simulink model "vehicle_motion_model_final_temp"  (R2021b)
settings: Solver=ode5  StartTime=0.0  StopTime=600  FixedStep=0.001  RelTol=1e-3
StopFcn:
  | % stop simulation callback function
  | figure(1);
  | out.x_gt.data = permute(out.x_gt.data,[3, 1, 2]);
  | plot3(out.x_gt.data(:, 1), out.x_gt.data(:, 2), -out.x_gt.data(:, 3), 'Color', 'r', 'LineWidth', 1.5);
  | legend('Истинная траектория')
  | xlabel('X, \itм');
  | ylabel('Y, \itм');
  | zlabel('Z, \itм');
  | figure(2);
  | plot3(out.x.data(:, 1), out.x.data(:, 2), -out.x.data(:, 3), 'Color', 'b', 'LineWidth', 1.5);
  | hold on;
  | xlabel('X, \itм');
  | ylabel('Y, \itм');
  | zlabel('Z, \itм');
  | % legend('pos')
  | hold on;
  | plot3(out.x_gt.data(:, 1), out.x_gt.data(:, 2), -out.x_gt.data(:, 3), 'Color', 'r', 'LineWidth', 1.5);
  | hold on;
  | legend('Рассчитанная траектория', 'Истинная траектория')
  | % errors
  | figure(3);
  | yyaxis left;
  | plot(out.hor_err_fus.time, out.hor_err_fus.data, 'Color', 'b', 'LineWidth', 1.5);
  | xlabel('время, \itс');
  | ylabel('Горизонтальная ошибка, \itм');
  | hold on;
  | yyaxis right;
  | plot(out.ver_err_fus.time, out.ver_err_fus.data, 'Color', 'r', 'LineWidth', 1.5);
  | ylabel('Вертикальная ошибка, \itм');
  | legend('Горизонтальная позиционная ошибка', 'Вертикальная позиционная ошибка');
  | grid on;
  | figure(4);
  | yyaxis left;
  | plot(out.hor_err_ins.time, out.hor_err_ins.data, '-', 'Color', 'b', 'LineWidth', 1.5);
  | xlabel('время, \itс');
  | ylabel('Горизонтальная ошибка, \itм');
  | hold on;
  | yyaxis right;
  | plot(out.ver_err_ins.time, out.ver_err_ins.data, '-', 'Color', 'r', 'LineWidth', 1.5);
  | ylabel('Вертикальная ошибка, \itм');
  | legend('Горизонтальная позиционная ошибка', 'Вертикальная позиционная ошибка');
  | grid on;
model workspace (MAT data in the model file):
  AxlIxx = 62.3745166667
  AxlM = 160
  Cps = 2
  CzWhlAxl = 557955.087061
  DCT_Param : object (value not decoded)
  Downshift_Speeds = [9.5625 12.9375 16.3125 19.6875 23.0625 26.4375 29.8125 33.1875 36.5625 39.9375 43.3125 46.6875 ... (28 elements, 4x7)]
  F0zWhlAxl = 16132.2380068
  HTCH : object (value not decoded)
  Hmax = 0.25
  KzWhlAxl = 58428920.0848
  NCyl = 6
  Pedal_Positions = [0.1 0.4 0.5 0.9]
  Pstd = 101325
  Q = [1  0  0; 0  1  0; 0  0  1]
  Rair = 287
  SUS : object (value not decoded)
  TRA : object (value not decoded)
  Trans : object (value not decoded)
  Tstd = 293.15
  Upshift_Speeds = [12.9375 16.3125 19.6875 33 26.4375 29.8125 33.1875 52.5 39.9375 43.3125 46.6875 77.25 ... (28 elements, 4x7)]
  VEH : object (value not decoded)
  Vd = 0.00346
  WH : Mass (value not decoded)
  dt3D = 0.05
  f_air = [0 0 0 0 0 0 0 0 0 0 0 0 ... (256 elements, 16x16)]
  f_co = [0 0 0 0 0 0 0 0 0 0 0 0 ... (256 elements, 16x16)]
  f_co2 = [0 0 0 0 0 0 0 0 0 0 0 0 ... (256 elements, 16x16)]
  f_eff = [352.135682859 352.135682859 320.724378192 303.655312657 295.930136708 291.240087194 291.240271258 291.240312459 291.240275452 291.240198499 291.240100781 291.240018769 ... (256 elements, 16x16)]
  f_fuel = [0 0 0 0 0 0 0 0 0 0 0 0 ... (256 elements, 16x16)]
  f_hc = [0 0 0 0 0 0 0 0 0 0 0 0 ... (256 elements, 16x16)]
  f_nox = [0 0 0 0 0 0 0 0 0 0 0 0 ... (256 elements, 16x16)]
  f_pm = [0 0 0 0 0 0 0 0 0 0 0 0 ... (256 elements, 16x16)]
  f_susp_axl_bp = [1 2]
  f_susp_dz_bp = [-0.325022776267 -0.315022776267 -0.305022776267 -0.205022776267 -0.105022776267 -0.00502277626717 0.0949772237328 0.194977223733 0.204977223733 0.214977223733]
  f_susp_dzdot_bp = [-3 -0.3 -0.2 -0.1 0 0.1 0.2 0.3 3]
  f_susp_fmz = [-144070.391448 -93629.24037 -75929.1118915 -20630.5828179 -15385.48216 -10140.3815021 -4895.28084414 349.819813785 -31916.3973792 18437.6709544 -83996.1993354 -33555.0482577 ... (43920 elements, 10x9x61x2x4)]
  f_susp_geom = [0 0 0 0 0 0 0 0 0 0 0 0 ... (3660 elements, 10x61x2x3)]
  f_susp_strgdelta_bp = [-0.523598775598 -0.506145483078 -0.488692190558 -0.471238898038 -0.453785605519 -0.436332312999 -0.418879020479 -0.401425727959 -0.383972435439 -0.366519142919 -0.349065850399 -0.331612557879 ... (61 elements, 1x61)]
  f_tbrake = [0 76.8593923996 105.140482948 131.533638111 157.926793274 176.658631717 176.65727296 176.656856686 176.656879077 176.657093756 176.657404516 176.65772406 ... (256 elements, 16x16)]
  f_tbrake_n_bpt = [0 649.519052838 912.419621844 1175.32019085 1438.22075986 1701.12132886 1964.02189787 2226.92246687 2489.82303588 2752.72360489 3015.62417389 3278.5247429 ... (16 elements, 1x16)]
  f_tbrake_t_bpt = [0 34.6410161514 61.0341713143 87.4273264773 113.82048164 140.213636803 166.606791966 192.999947129 219.393102292 245.786257455 272.179412618 298.572567781 ... (16 elements, 1x16)]
  f_texh = [766.752464599 766.752464599 786.17542386 801.679939032 884.591982581 910.574397722 910.571871054 910.570774534 910.570601632 910.570821151 910.571247242 910.571639815 ... (256 elements, 16x16)]
  f_twc_eff_co = [0.17 0.25 0.45 0.99 0.99 0.99 0.99]
  f_twc_eff_hc = [0.21 0.375 0.75 0.98 0.98 0.98 0.98]
  f_twc_eff_lam = [0.909090909 0.944055944 0.979020979 1 1.013986014 1.048951049 1.083916084]
  f_twc_eff_nox = [0.98 0.98 0.98 0.97 0.05 0.02 0]
  h = 0.134
symbols that are objects in the model workspace (value not decoded): VEH
libraries: aerolibcommonsys x8, sharedtransform x8, sharedutil x7, autolibsharedcommon x7, autolibutils x4, vehdynlibtirecommon x3, dspstat3 x2, mspsensorlib x1, aerolibnav x1, shared6dof x1, autolibshared x1, vehdynlibsuspension x1
(part 5 of 9)

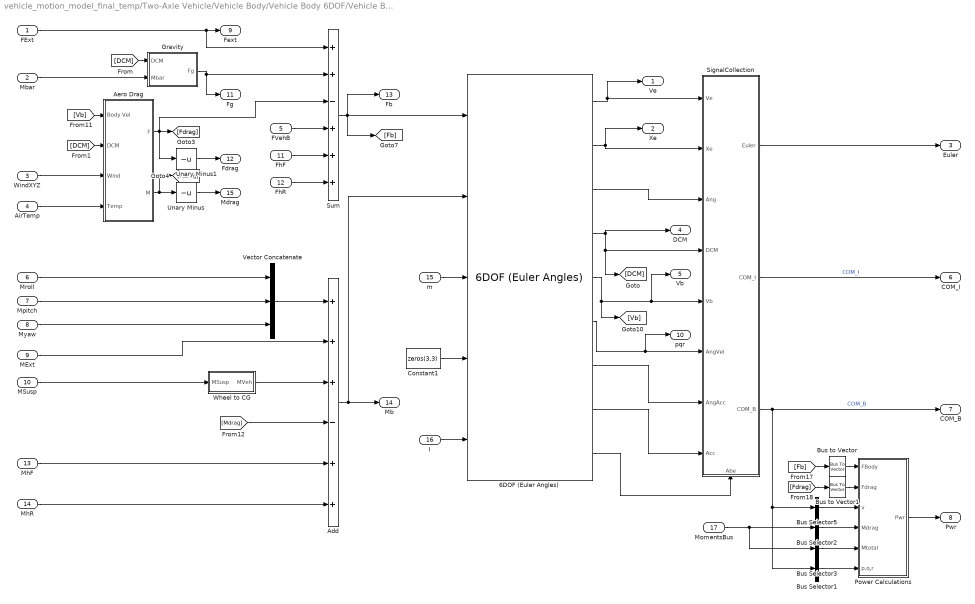
== system vehicle_motion_model_final_temp/Two-Axle Vehicle/Vehicle Body/Vehicle Body 6DOF/Vehicle Body 6DOF/6 DOF Generic Vehicle Body ==
  FExt : Inport  Unit=N
  Mbar : Inport  Port=2
  WindXYZ : Inport  Port=3  Unit=m/s
  AirTemp : Inport  Port=4  Unit=K
  FVehB : Inport  Port=5
  Mroll : Inport  Port=6
  Mpitch : Inport  Port=7
  Myaw : Inport  Port=8
  MExt : Inport  Port=9  Unit=N*m
  MSusp : Inport  Port=10  Unit=N*m
  FhF : Inport  Port=11  Unit=N
  FhR : Inport  Port=12  Unit=N
  MhF : Inport  Port=13  Unit=N*m
  MhR : Inport  Port=14  Unit=N*m
  m : Inport  Port=15
  I : Inport  Port=16
  MomentsBus : Inport  Port=17  Unit=N*m
  6DOF (Euler Angles) : shared6dof/6DOF (Euler Angles)  units=Metric (MKS)  mtype=Custom Variable  rep=Euler Angles  xme_0=Xe_o  Vm_0=xbdot_o  eul_0=eul_o  pm_0=p_o  mass_0=m  mass_e=[0 0 0]  mass_f=[0 0 0]  inertia=Iveh  inertia_e=[0 0 0]  inertia_f=[0 0 0]  k_quat=[0 0 0]  vre_flag=off  abi_flag=on  aMode=2  xme_statename=''  Vm_statename=''  eul_statename=''  quat_statename=''  pm_statename=''  mass_statename=''
      settings: SourceProductBaseCode=AE,PW,DR,MT,UV,VE
  Add : Sum  Inputs=+++-++
  Aero Drag : Subsystem
  Bus Selector1 : BusSelector  OutputSignals=AngVel.p,AngVel.q,AngVel.r  OutputAsBus=on
  Bus Selector2 : BusSelector  OutputSignals=Drag.Mx,Drag.My,Drag.Mz  OutputAsBus=on
  Bus Selector3 : BusSelector  OutputSignals=Body.Mx,Body.My,Body.Mz  OutputAsBus=on
  Bus Selector5 : BusSelector  OutputSignals=Vel.xdot,Vel.ydot,Vel.zdot  OutputAsBus=on
  Bus to Vector : BusToVector
  Bus to Vector1 : BusToVector
  Constant1 : Constant  Value=zeros(3,3)
  Gravity : Subsystem
  Power Calculations : Subsystem  VariantControl=2
  SignalCollection : Subsystem
      settings: PortSchema="{\"entries\":[{\"content\":{\"sides\":[{\"content\":{\"connectorIds\":[\"In1\",\"In2\",\"In3\",\"In4\",\"In5\",\"In6\",\"In7\",\"In8\"]},\"type\":\"ConnectorPlacement.EquallySpacedRectSide\",\"uuid\":\"876487b8-56e9-4112-b104-05c1a2771af8\"},{\"content\":{\"connectorIds\":[\"Out1\",\"Out2\",\"Out3\"],\"side\":\"RIGHT\"},\"type\":\"ConnectorPlacement.EquallySpacedRectSide\",\"uuid\":\"0e979842-5463-4993-8b9a-4ed5d1e46013\"},{\"content\":{\"connectorIds\":[],\"side\":\"TOP\"},\"type\":\"ConnectorPlacement.EquallySpacedRectSide\",\"uuid\":\"9909ba18-debd-4c28-8048-279359011dab\"},{\"content\":{\"connectorIds\":[\"In9\"],\"side\":\"BOTTOM\"},\"type\":\"ConnectorPlacement.EquallySpacedRectSide\",\"uuid\":\"e172f998-bdb6-4b24-8333-70df8a68a329\"}]},\"type\":\"ConnectorPlacement.EquallySpacedConnector\",\"uuid\":\"1f4bc3e0-d188-4108-8b40-be3dce1f4c41\"}],\"packageUris\":[\"http://schema.mathworks.com/mf0/Connector/R2020b\"],\"version\":\"1.0\"}"
  Sum : Sum  Inputs=++-+++  InputSameDT=on  SaturateOnIntegerOverflow=on  OutDataTypeStr=Inherit: Same as first input
  Unary Minus : UnaryMinus
  Unary Minus1 : UnaryMinus
  Vector Concatenate : Concatenate  NumInputs=3
  Wheel to CG : Subsystem
  Ve : Outport  Unit=m/s  VectorParamsAs1DForOutWhenUnconnected=off
  Xe : Outport  Port=2  Unit=m  VectorParamsAs1DForOutWhenUnconnected=off
  Euler : Outport  Port=3  Unit=rad  VectorParamsAs1DForOutWhenUnconnected=off
  DCM : Outport  Port=4  VectorParamsAs1DForOutWhenUnconnected=off
  Vb : Outport  Port=5  Unit=m/s  VectorParamsAs1DForOutWhenUnconnected=off
  COM_I : Outport  Port=6  VectorParamsAs1DForOutWhenUnconnected=off
  COM_B : Outport  Port=7  VectorParamsAs1DForOutWhenUnconnected=off
  Pwr : Outport  Port=8  VectorParamsAs1DForOutWhenUnconnected=off
  Fext : Outport  Port=9  VectorParamsAs1DForOutWhenUnconnected=off
  pqr : Outport  Port=10  Unit=rad/s  VectorParamsAs1DForOutWhenUnconnected=off
  Fg : Outport  Port=11  VectorParamsAs1DForOutWhenUnconnected=off
  Fdrag : Outport  Port=12  VectorParamsAs1DForOutWhenUnconnected=off
  Fb : Outport  Port=13  VectorParamsAs1DForOutWhenUnconnected=off
  Mb : Outport  Port=14  VectorParamsAs1DForOutWhenUnconnected=off
  Mdrag : Outport  Port=15  VectorParamsAs1DForOutWhenUnconnected=off
  wires:
  6DOF (Euler Angles)/9 -> SignalCollection/9(Abe)
  Unary Minus1/1 -> Fdrag/1
  Unary Minus/1 -> Mdrag/1
  MomentsBus/1 -> Bus Selector2/1, Bus Selector3/1
  MhR/1 -> Add/6
  FhR/1 -> Sum/6
  FhF/1 -> Sum/5
  MhF/1 -> Add/5
  Mbar/1 -> Gravity/2(Mbar)
  I/1 -> 6DOF (Euler Angles)/5
  Mpitch/1 -> Vector Concatenate/2
  Myaw/1 -> Vector Concatenate/3
  Bus Selector3/1 -> Power Calculations/5(Mtotal)
  SignalCollection/1(Euler) -> Euler/1
  [Mdrag] -> Add/4
  Bus to Vector/1 -> Power Calculations/1(FBody)
  Power Calculations/1(Pwr) -> Pwr/1
  6DOF (Euler Angles)/2 -> Xe/1, SignalCollection/2(Xe)
  AirTemp/1 -> Aero Drag/4(Temp)
  [Fdrag] -> Bus to Vector1/1
  Vector Concatenate/1 -> Add/1
  MExt/1 -> Add/2
  6DOF (Euler Angles)/6 -> SignalCollection/6(AngVel), pqr/1
  6DOF (Euler Angles)/5 -> SignalCollection/5(Vb), Vb/1, [Vb]
  FExt/1 -> Fext/1, Sum/1
  6DOF (Euler Angles)/4 -> DCM/1, SignalCollection/4(DCM), [DCM]
  MSusp/1 -> Wheel to CG/1(MSusp)
  FVehB/1 -> Sum/4
  [DCM] -> Aero Drag/2(DCM)
  SignalCollection/2(COM_I) -> COM_I/1  "COM_I"
  WindXYZ/1 -> Aero Drag/3(Wind)
  [Vb] -> Aero Drag/1(Body Vel)
  Gravity/1(Fg) -> Sum/2, Fg/1
  [DCM] -> Gravity/1(DCM)
  Aero Drag/2(M) -> [Mdrag], Unary Minus/1
  6DOF (Euler Angles)/3 -> SignalCollection/3(Ang)
  Bus Selector5/1 -> Power Calculations/3(v)
  Sum/1 -> 6DOF (Euler Angles)/1, [Fb], Fb/1
  Mroll/1 -> Vector Concatenate/1
  6DOF (Euler Angles)/8 -> SignalCollection/8(Acc)
  Wheel to CG/1(MVeh) -> Add/3
  6DOF (Euler Angles)/7 -> SignalCollection/7(AngAcc)
  Bus to Vector1/1 -> Power Calculations/2(Fdrag)
  m/1 -> 6DOF (Euler Angles)/3
  [Fb] -> Bus to Vector/1
  SignalCollection/3(COM_B) -> Bus Selector5/1, Bus Selector1/1, COM_B/1  "COM_B"
  Add/1 -> Mb/1, 6DOF (Euler Angles)/2
  6DOF (Euler Angles)/1 -> Ve/1, SignalCollection/1(Ve)
  Constant1/1 -> 6DOF (Euler Angles)/4
  Bus Selector2/1 -> Power Calculations/4(Mdrag)
  Bus Selector1/1 -> Power Calculations/6(p,q,r)
  Aero Drag/1(F) -> Sum/3, [Fdrag], Unary Minus1/1

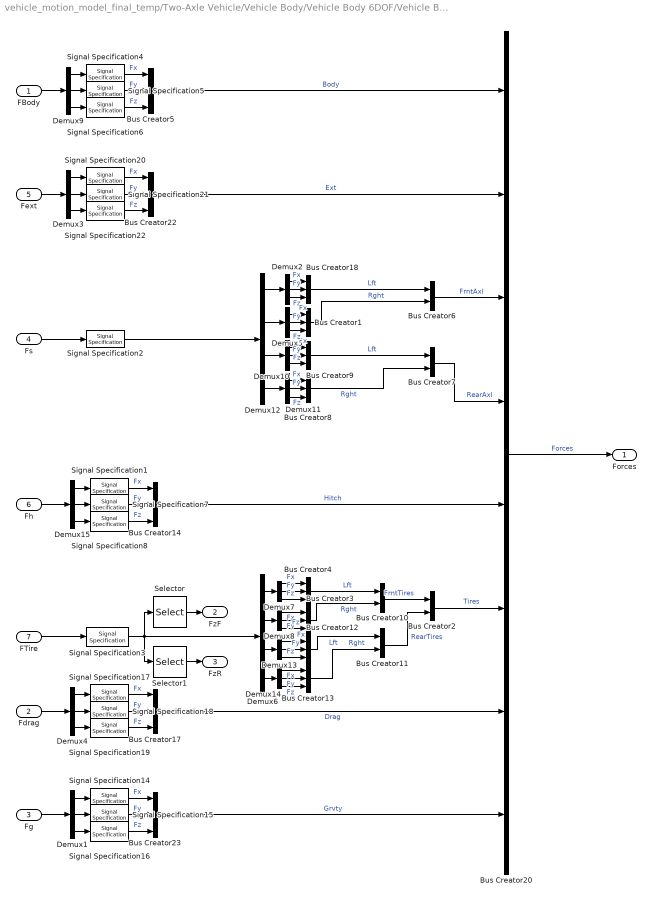
== system vehicle_motion_model_final_temp/Two-Axle Vehicle/Vehicle Body/Vehicle Body 6DOF/Vehicle Body 6DOF/Forces ==
  FBody : Inport
  Fdrag : Inport  Port=2
  Fg : Inport  Port=3
  Fs : Inport  Port=4  Unit=N
  Fext : Inport  Port=5
  Fh : Inport  Port=6
  FTire : Inport  Port=7
  Bus Creator{1,3..5,8..9,12..14,17..18,22..23} (13 alike) : BusCreator  Inputs=3
  Bus Creator{2,6..7,10..11} (5 alike) : BusCreator  Inputs=2
  Bus Creator20 : BusCreator  Inputs=8
  Demux{1..5,7..11,13..15} (13 alike) : Demux  Outputs=3
  Demux12 : Demux  Outputs=[3,3,3,3]
  Demux6 : Demux  Outputs=[3,3,3,3]
  Selector : Selector  InputPortWidth=12  IndexOptions=Index vector (dialog)  Indices=[3,6]  OutputSizes=1
  Selector1 : Selector  InputPortWidth=12  IndexOptions=Index vector (dialog)  Indices=[9,12]  OutputSizes=1
  Signal Specification{1..8,14..22} (17 alike) : SignalSpecification  Unit=N
  Forces : Outport  VectorParamsAs1DForOutWhenUnconnected=off
  FzF : Outport  Port=2  VectorParamsAs1DForOutWhenUnconnected=off
  FzR : Outport  Port=3  VectorParamsAs1DForOutWhenUnconnected=off
  wires:
  Bus Creator14/1 -> Bus Creator20/5  "Hitch"
  Fh/1 -> Demux15/1
  Demux15/3 -> Signal Specification8/1
  Demux15/2 -> Signal Specification7/1
  Demux15/1 -> Signal Specification1/1
  Signal Specification7/1 -> Bus Creator14/2  "Fy"
  Signal Specification1/1 -> Bus Creator14/1  "Fx"
  Signal Specification8/1 -> Bus Creator14/3  "Fz"
  Selector1/1 -> FzR/1
  Selector/1 -> FzF/1
  Demux13/3 -> Bus Creator12/3  "Fz"
  Bus Creator13/1 -> Bus Creator11/2  "Rght"
  Demux14/1 -> Bus Creator13/1  "Fx"
  Demux14/2 -> Bus Creator13/2  "Fy"
  Demux14/3 -> Bus Creator13/3  "Fz"
  Demux6/4 -> Demux14/1
  Demux6/3 -> Demux13/1
  Demux13/2 -> Bus Creator12/2  "Fy"
  Demux13/1 -> Bus Creator12/1  "Fx"
  Signal Specification2/1 -> Demux12/1
  Bus Creator12/1 -> Bus Creator11/1  "Lft"
  Bus Creator3/1 -> Bus Creator10/2  "Rght"
  Bus Creator4/1 -> Bus Creator10/1  "Lft"
  Demux12/3 -> Demux10/1
  Demux12/4 -> Demux11/1
  Demux11/1 -> Bus Creator8/1  "Fx"
  Demux11/2 -> Bus Creator8/2  "Fy"
  Demux11/3 -> Bus Creator8/3  "Fz"
  Demux10/3 -> Bus Creator9/3  "Fz"
  Demux10/2 -> Bus Creator9/2  "Fy"
  Demux10/1 -> Bus Creator9/1  "Fx"
  Bus Creator9/1 -> Bus Creator7/1  "Lft"
  Bus Creator8/1 -> Bus Creator7/2  "Rght"
  Bus Creator1/1 -> Bus Creator6/2  "Rght"
  Bus Creator18/1 -> Bus Creator6/1  "Lft"
  Demux1/1 -> Signal Specification14/1
  Fg/1 -> Demux1/1
  Demux1/3 -> Signal Specification16/1
  Demux1/2 -> Signal Specification15/1
  Bus Creator23/1 -> Bus Creator20/8  "Grvty"
  Bus Creator20/1 -> Forces/1  "Forces"
  Signal Specification16/1 -> Bus Creator23/3  "Fz"
  Signal Specification19/1 -> Bus Creator17/3  "Fz"
  Signal Specification14/1 -> Bus Creator23/1  "Fx"
  Signal Specification17/1 -> Bus Creator17/1  "Fx"
  Signal Specification18/1 -> Bus Creator17/2  "Fy"
  Signal Specification21/1 -> Bus Creator22/2  "Fy"
  Signal Specification15/1 -> Bus Creator23/2  "Fy"
  Signal Specification20/1 -> Bus Creator22/1  "Fx"
  Signal Specification22/1 -> Bus Creator22/3  "Fz"
  Bus Creator22/1 -> Bus Creator20/2  "Ext"
  Fext/1 -> Demux3/1
  Demux3/1 -> Signal Specification20/1
  Demux3/2 -> Signal Specification21/1
  Demux3/3 -> Signal Specification22/1
  Demux4/1 -> Signal Specification17/1
  Demux4/2 -> Signal Specification18/1
  Demux4/3 -> Signal Specification19/1
  Fdrag/1 -> Demux4/1
  Bus Creator6/1 -> Bus Creator20/3  "FrntAxl"
  Bus Creator7/1 -> Bus Creator20/4  "RearAxl"
  Demux2/1 -> Bus Creator18/1  "Fx"
  Demux2/2 -> Bus Creator18/2  "Fy"
  Demux2/3 -> Bus Creator18/3  "Fz"
  Demux5/3 -> Bus Creator1/3  "Fz"
  Demux5/2 -> Bus Creator1/2  "Fy"
  Demux8/1 -> Bus Creator3/1  "Fx"
  Demux8/2 -> Bus Creator3/2  "Fy"
  Demux8/3 -> Bus Creator3/3  "Fz"
  Demux7/3 -> Bus Creator4/3  "Fz"
  Demux7/2 -> Bus Creator4/2  "Fy"
  Demux7/1 -> Bus Creator4/1  "Fx"
  Bus Creator11/1 -> Bus Creator2/2  "RearTires"
  Bus Creator10/1 -> Bus Creator2/1  "FrntTires"
  Demux5/1 -> Bus Creator1/1  "Fx"
  Fs/1 -> Signal Specification2/1
  Demux12/2 -> Demux5/1
  Demux12/1 -> Demux2/1
  FTire/1 -> Signal Specification3/1
  Signal Specification3/1 -> Demux6/1, Selector/1, Selector1/1
  Demux6/1 -> Demux7/1
  Demux6/2 -> Demux8/1
  Bus Creator2/1 -> Bus Creator20/6  "Tires"
  Bus Creator17/1 -> Bus Creator20/7  "Drag"
  Bus Creator5/1 -> Bus Creator20/1  "Body"
  Demux9/3 -> Signal Specification6/1
  Demux9/2 -> Signal Specification5/1
  Demux9/1 -> Signal Specification4/1
  FBody/1 -> Demux9/1
  Signal Specification6/1 -> Bus Creator5/3  "Fz"
  Signal Specification4/1 -> Bus Creator5/1  "Fx"
  Signal Specification5/1 -> Bus Creator5/2  "Fy"

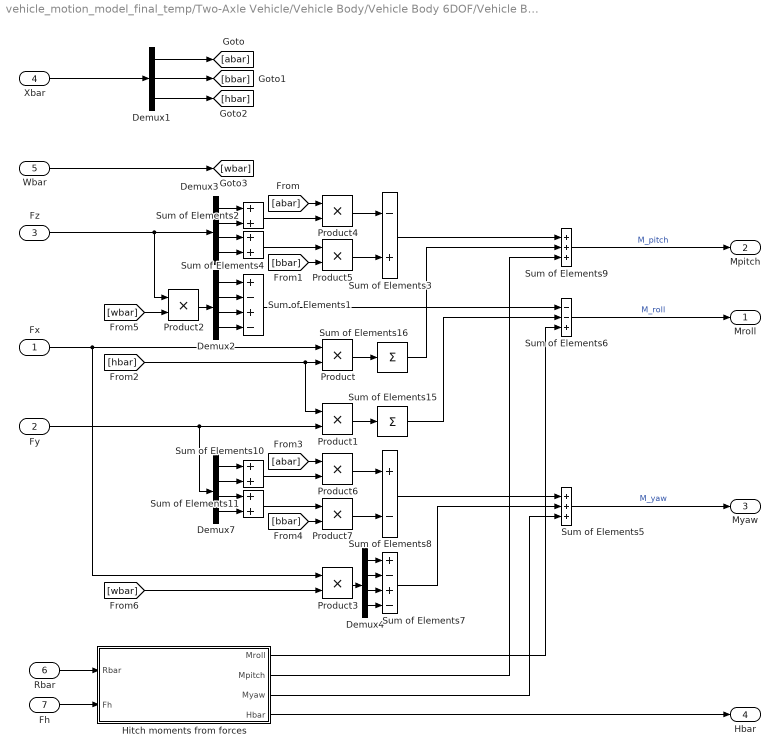
== system vehicle_motion_model_final_temp/Two-Axle Vehicle/Vehicle Body/Vehicle Body 6DOF/Vehicle Body 6DOF/Moment Calc ==
  Fx : Inport
  Fy : Inport  Port=2
  Fz : Inport  Port=3
  Xbar : Inport  Port=4
  Wbar : Inport  Port=5
  Rbar : Inport  Port=6
  Fh : Inport  Port=7
  Demux1 : Demux  Outputs=3
  Demux{2..4,7} (4 alike) : Demux
  Hitch moments from forces : Subsystem
  Product{,1..7} (8 alike) : Product
  Sum of Elements1 : Sum  Inputs=+-+-
  Sum of Elements{2,4,10..11} (4 alike) : Sum
  Sum of Elements15 : Sum  Inputs=+
  Sum of Elements16 : Sum  Inputs=+
  Sum of Elements3 : Sum  Inputs=-+
  Sum of Elements5 : Sum  Inputs=+++
  Sum of Elements6 : Sum  Inputs=--+
  Sum of Elements7 : Sum  Inputs=+-+-
  Sum of Elements8 : Sum  Inputs=+-
  Sum of Elements9 : Sum  Inputs=+++
  Mroll : Outport  VectorParamsAs1DForOutWhenUnconnected=off
  Mpitch : Outport  Port=2  VectorParamsAs1DForOutWhenUnconnected=off
  Myaw : Outport  Port=3  VectorParamsAs1DForOutWhenUnconnected=off
  Hbar : Outport  Port=4  VectorParamsAs1DForOutWhenUnconnected=off
  wires:
  Hitch moments from forces/4(Hbar) -> Hbar/1
  Fh/1 -> Hitch moments from forces/2(Fh)
  Hitch moments from forces/3(Myaw) -> Sum of Elements5/3
  Hitch moments from forces/2(Mpitch) -> Sum of Elements9/3
  Hitch moments from forces/1(Mroll) -> Sum of Elements6/3
  Rbar/1 -> Hitch moments from forces/1(Rbar)
  Wbar/1 -> [wbar]
  Demux1/1 -> [abar]
  Demux1/2 -> [bbar]
  [wbar] -> Product2/2
  Xbar/1 -> Demux1/1
  Demux1/3 -> [hbar]
  Demux7/2 -> Sum of Elements10/2
  Demux7/1 -> Sum of Elements10/1
  Demux7/4 -> Sum of Elements11/2
  Demux7/3 -> Sum of Elements11/1
  Product6/1 -> Sum of Elements8/1
  Product7/1 -> Sum of Elements8/2
  Sum of Elements11/1 -> Product7/1
  Sum of Elements10/1 -> Product6/2
  [abar] -> Product6/1
  [bbar] -> Product7/2
  [bbar] -> Product5/2
  [abar] -> Product4/1
  [wbar] -> Product3/2
  Product3/1 -> Demux4/1
  Demux4/3 -> Sum of Elements7/3
  Demux4/2 -> Sum of Elements7/2
  Product2/1 -> Demux2/1
  Demux2/3 -> Sum of Elements1/3
  Demux2/2 -> Sum of Elements1/2
  Fy/1 -> Product1/2, Demux7/1
  Demux4/1 -> Sum of Elements7/1
  Demux4/4 -> Sum of Elements7/4
  Demux2/4 -> Sum of Elements1/4
  Fx/1 -> Product/1, Product3/1
  Fz/1 -> Demux3/1, Product2/1
  Sum of Elements1/1 -> Sum of Elements6/1
  Sum of Elements2/1 -> Product4/2
  Sum of Elements4/1 -> Product5/1
  Demux3/3 -> Sum of Elements4/1
  Sum of Elements3/1 -> Sum of Elements9/1
  [hbar] -> Product/2, Product1/1
  Demux3/4 -> Sum of Elements4/2
  Demux3/1 -> Sum of Elements2/1
  Demux3/2 -> Sum of Elements2/2
  Sum of Elements15/1 -> Sum of Elements6/2
  Sum of Elements8/1 -> Sum of Elements5/1
  Sum of Elements5/1 -> Myaw/1  "M_yaw"
  Sum of Elements16/1 -> Sum of Elements9/2
  Product5/1 -> Sum of Elements3/2
  Sum of Elements7/1 -> Sum of Elements5/2
  Demux2/1 -> Sum of Elements1/1
  Product4/1 -> Sum of Elements3/1
  Sum of Elements9/1 -> Mpitch/1  "M_pitch"
  Sum of Elements6/1 -> Mroll/1  "M_roll"
  Product/1 -> Sum of Elements16/1
  Product1/1 -> Sum of Elements15/1

== system vehicle_motion_model_final_temp/Two-Axle Vehicle/Vehicle Body/Vehicle Body 6DOF/Vehicle Body 6DOF/Moments ==
  MBody : Inport
  Mdrag : Inport  Port=2
  MExt : Inport  Port=3
  Mh : Inport  Port=4
  Bus Creator{1..3,24} (4 alike) : BusCreator  Inputs=3
  Bus Creator7 : BusCreator  Inputs=4
  Demux{,1..3} (4 alike) : Demux  Outputs=3
  Signal Specification{1..11,23} (12 alike) : SignalSpecification  Unit=N*m
  Moments : Outport  VectorParamsAs1DForOutWhenUnconnected=off
  wires:
  Mh/1 -> Demux3/1
  Demux3/3 -> Signal Specification10/1
  Demux3/1 -> Signal Specification11/1
  Demux3/2 -> Signal Specification9/1
  Signal Specification11/1 -> Bus Creator2/1  "Mx"
  Bus Creator2/1 -> Bus Creator7/4  "Hitch"
  Signal Specification9/1 -> Bus Creator2/2  "My"
  Signal Specification10/1 -> Bus Creator2/3  "Mz"
  Signal Specification23/1 -> Bus Creator24/1  "Mx"
  Bus Creator24/1 -> Bus Creator7/1  "Body"
  Signal Specification1/1 -> Bus Creator24/2  "My"
  Signal Specification2/1 -> Bus Creator24/3  "Mz"
  Bus Creator1/1 -> Bus Creator7/2  "Drag"
  Bus Creator7/1 -> Moments/1  "Moments"
  Demux/2 -> Signal Specification1/1
  Demux/1 -> Signal Specification23/1
  Demux/3 -> Signal Specification2/1
  MBody/1 -> Demux/1
  Mdrag/1 -> Demux1/1
  Demux1/3 -> Signal Specification4/1
  Demux1/1 -> Signal Specification5/1
  Demux1/2 -> Signal Specification3/1
  Signal Specification4/1 -> Bus Creator1/3  "Mz"
  Signal Specification3/1 -> Bus Creator1/2  "My"
  Signal Specification5/1 -> Bus Creator1/1  "Mx"
  MExt/1 -> Demux2/1
  Signal Specification7/1 -> Bus Creator3/3  "Mz"
  Signal Specification6/1 -> Bus Creator3/2  "My"
  Bus Creator3/1 -> Bus Creator7/3  "Ext"
  Signal Specification8/1 -> Bus Creator3/1  "Mx"
  Demux2/2 -> Signal Specification6/1
  Demux2/1 -> Signal Specification8/1
  Demux2/3 -> Signal Specification7/1

== system vehicle_motion_model_final_temp/Two-Axle Vehicle/Vehicle Body/Vehicle Body 6DOF/Vehicle Body 6DOF/Signal Routing ==
  InertCg : Inport
  BdyFrmCg : Inport  Port=2
  Power : Inport  Port=3
  Hbar : Inport  Port=4
  Rbar : Inport  Port=5
  HPbar : Inport  Port=6
  Forces : Inport  Port=7
  Moments : Inport  Port=8
  Bus Creator1 : BusCreator  Inputs=8
  Bus Creator2 : BusCreator  Inputs=5
  Bus Creator{3..6} (4 alike) : BusCreator  Inputs=2
  Hard Point Coordinate Transform Front Left : Subsystem
  Hard Point Coordinate Transform Front Right : Subsystem
  Hard Point Coordinate Transform Geometric : Subsystem
  Hard Point Coordinate Transform Hitch : Subsystem
  Hard Point Coordinate Transform Rear Left : Subsystem
  Hard Point Coordinate Transform Rear Right : Subsystem
  InertFrm : Outport  VectorParamsAs1DForOutWhenUnconnected=off
  BdyFrm : Outport  Port=2  VectorParamsAs1DForOutWhenUnconnected=off
  wires:
  Hbar/1 -> Hard Point Coordinate Transform Hitch/3(Hbar)
  Hard Point Coordinate Transform Hitch/2(Body) -> Bus Creator1/6  "Hitch"
  Hard Point Coordinate Transform Hitch/1(Inert) -> Bus Creator2/4  "Hitch"
  Rbar/1 -> Hard Point Coordinate Transform Geometric/3(Rbar)
  HPbar/1 -> Hard Point Coordinate Transform Front Left/3(HPbar), Hard Point Coordinate Transform Rear Left/3(HPbar), Hard Point Coordinate Transform Rear Right/3(HPbar), Hard Point Coordinate Transform Front Right/3(HPbar)
  Bus Creator6/1 -> Bus Creator1/5  "RearAxl"
  Hard Point Coordinate Transform Front Left/2(Body) -> Bus Creator5/1  "Lft"
  Hard Point Coordinate Transform Front Right/2(Body) -> Bus Creator5/2  "Rght"
  Hard Point Coordinate Transform Rear Left/2(Body) -> Bus Creator6/1  "Lft"
  Hard Point Coordinate Transform Rear Right/2(Body) -> Bus Creator6/2  "Rght"
  Hard Point Coordinate Transform Rear Right/1(Inert) -> Bus Creator4/2  "Rght"
  Hard Point Coordinate Transform Rear Left/1(Inert) -> Bus Creator4/1  "Lft"
  Hard Point Coordinate Transform Front Right/1(Inert) -> Bus Creator3/2  "Rght"
  Hard Point Coordinate Transform Front Left/1(Inert) -> Bus Creator3/1  "Lft"
  Moments/1 -> Bus Creator1/3  "Moments"
  Bus Creator5/1 -> Bus Creator1/4  "FrntAxl"
  InertCg/1 -> Bus Creator2/1, Hard Point Coordinate Transform Front Left/1(InertFrmCg), Hard Point Coordinate Transform Front Right/1(InertFrmCg), Hard Point Coordinate Transform Geometric/1(InertFrmCg), Hard Point Coordinate Transform Hitch/1(InertFrmCg), Hard Point Coordinate Transform Rear Right/1(InertFrmCg), Hard Point Coordinate Transform Rear Left/1(InertFrmCg)  "Cg"
  Bus Creator4/1 -> Bus Creator2/3  "RearAxl"
  Bus Creator2/1 -> InertFrm/1  "InertFrm"
  Bus Creator1/1 -> BdyFrm/1  "BdyFrm"
  Bus Creator3/1 -> Bus Creator2/2  "FrntAxl"
  BdyFrmCg/1 -> Hard Point Coordinate Transform Front Left/2(BdyFrmCg), Hard Point Coordinate Transform Front Right/2(BdyFrmCg), Hard Point Coordinate Transform Rear Left/2(BdyFrmCg), Hard Point Coordinate Transform Rear Right/2(BdyFrmCg), Hard Point Coordinate Transform Geometric/2(BdyFrmCg), Bus Creator1/1, Hard Point Coordinate Transform Hitch/2(BdyFrmCg)  "Cg"
  Forces/1 -> Bus Creator1/2  "Forces"
  Power/1 -> Bus Creator1/7  "Pwr"
  Hard Point Coordinate Transform Geometric/2(Body) -> Bus Creator1/8  "Geom"
  Hard Point Coordinate Transform Geometric/1(Inert) -> Bus Creator2/5  "Geom"

== system vehicle_motion_model_final_temp/Two-Axle Vehicle/Vehicle Body/Vehicle Body 6DOF/Vehicle Body 6DOF/Susp2Chassis ==
  F : Inport
  Reshape : Reshape  OutputDimensionality=Customize  OutputDimensions=[3,4]
  Reshape1 : Reshape
  Reshape2 : Reshape
  Reshape3 : Reshape
  Selector1 : Selector  NumberOfDimensions=2  InputPortWidth=3  IndexOptions=Index vector (dialog),Select all  Indices=[1],1  OutputSizes=1,1
  Selector2 : Selector  NumberOfDimensions=2  InputPortWidth=3  IndexOptions=Index vector (dialog),Select all  Indices=[2],1  OutputSizes=1,1
  Selector3 : Selector  NumberOfDimensions=2  InputPortWidth=3  IndexOptions=Index vector (dialog),Select all  Indices=[3],1  OutputSizes=1,1
  Selector4 : Selector  NumberOfDimensions=2  InputPortWidth=3  IndexOptions=Select all,Index vector (dialog)  Indices=[1],2  OutputSizes=1,1
  Selector5 : Selector  NumberOfDimensions=2  InputPortWidth=3  IndexOptions=Select all,Index vector (dialog)  Indices=[1],3  OutputSizes=1,1
  Selector6 : Selector  NumberOfDimensions=2  InputPortWidth=3  IndexOptions=Select all,Index vector (dialog)  Indices=[1],4  OutputSizes=1,1
  Selector7 : Selector  NumberOfDimensions=2  InputPortWidth=3  IndexOptions=Select all,Index vector (dialog)  Indices=[1],1  OutputSizes=1,1
  Sum of Elements : Sum  Inputs=+
  Sum of Elements1 : Sum  Inputs=+
  Sum of Elements2 : Sum  Inputs=+
  Vector Concatenate : Concatenate  NumInputs=3
  Vector Concatenate2 : Concatenate  NumInputs=4
  Fs : Outport  VectorParamsAs1DForOutWhenUnconnected=off
  FVehB : Outport  Port=2  VectorParamsAs1DForOutWhenUnconnected=off
  FxW : Outport  Port=3  VectorParamsAs1DForOutWhenUnconnected=off
  FyW : Outport  Port=4  VectorParamsAs1DForOutWhenUnconnected=off
  FzW : Outport  Port=5  VectorParamsAs1DForOutWhenUnconnected=off
  wires:
  Reshape3/1 -> Sum of Elements2/1, FzW/1
  Reshape2/1 -> Sum of Elements1/1, FyW/1
  Reshape1/1 -> Sum of Elements/1, FxW/1
  Selector6/1 -> Vector Concatenate2/4
  Reshape/1 -> Selector7/1, Selector4/1, Selector5/1, Selector6/1, Selector1/1, Selector2/1, Selector3/1
  Selector5/1 -> Vector Concatenate2/3
  Selector7/1 -> Vector Concatenate2/1
  Selector4/1 -> Vector Concatenate2/2
  Vector Concatenate2/1 -> Fs/1
  Selector3/1 -> Reshape3/1
  Selector2/1 -> Reshape2/1
  Selector1/1 -> Reshape1/1
  Vector Concatenate/1 -> FVehB/1
  Sum of Elements2/1 -> Vector Concatenate/3
  Sum of Elements1/1 -> Vector Concatenate/2
  Sum of Elements/1 -> Vector Concatenate/1
  F/1 -> Reshape/1

== system vehicle_motion_model_final_temp/Two-Axle Vehicle/Wheels and Tires/Wheels and Tires/Tire2Veh/Routing ==
  <Mz> : Inport
  <Mx> : Inport  Port=2
  <My> : Inport  Port=3
  <Re> : Inport  Port=4
  <z> : Inport  Port=5
  <zdot> : Inport  Port=6
  <Kappa> : Inport  Port=7
  <Alpha> : Inport  Port=8
  Omega : Inport  Port=9
  Fx : Inport  Port=10
  Fy : Inport  Port=11
  Fz : Inport  Port=12
  Bus Creator : BusCreator  Inputs=12
  Reshape : Reshape  OutputDimensionality=Row vector (2-D)
  Reshape1 : Reshape  OutputDimensionality=Row vector (2-D)
  Unary Minus1 : UnaryMinus
  Unary Minus2 : UnaryMinus
  Out1 : Outport  VectorParamsAs1DForOutWhenUnconnected=off
  Out2 : Outport  Port=2  VectorParamsAs1DForOutWhenUnconnected=off
  Out3 : Outport  Port=3  VectorParamsAs1DForOutWhenUnconnected=off
  wires:
  <Re>/1 -> Bus Creator/8
  Unary Minus1/1 -> Reshape/1, Bus Creator/9  "z"
  Fz/1 -> Bus Creator/4
  <zdot>/1 -> Unary Minus2/1
  <Mz>/1 -> Bus Creator/7
  Unary Minus2/1 -> Reshape1/1, Bus Creator/10  "zdot"
  <z>/1 -> Unary Minus1/1
  Bus Creator/1 -> Out1/1
  Fy/1 -> Bus Creator/3
  Omega/1 -> Bus Creator/1  "Omega"
  Fx/1 -> Bus Creator/2
  Reshape1/1 -> Out3/1
  <Kappa>/1 -> Bus Creator/11
  Reshape/1 -> Out2/1
  <Mx>/1 -> Bus Creator/5
  <My>/1 -> Bus Creator/6
  <Alpha>/1 -> Bus Creator/12

== system vehicle_motion_model_final_temp/Two-Axle Vehicle/Wheels and Tires/Wheels and Tires/Tire2Veh/Subsystem1 ==
  Fin : Inport
  Demux : Demux
  Gain12 : Gain  Gain=VEH.NumberOfWheelsPerRearAxle
  Gain13 : Gain  Gain=VEH.NumberOfWheelsPerRearAxle
  Gain14 : Gain  Gain=1/2
  Gain8 : Gain  Gain=VEH.NumberOfWheelsPerFrontAxle
  Gain9 : Gain  Gain=VEH.NumberOfWheelsPerFrontAxle
  Mux1 : Mux
  Reshape : Reshape  OutputDimensionality=Column vector (2-D)
  Fout : Outport
  wires:
  Reshape/1 -> Fout/1
  Gain14/1 -> Reshape/1
  Demux/3 -> Gain12/1
  Demux/1 -> Gain8/1
  Demux/2 -> Gain9/1
  Gain8/1 -> Mux1/1
  Gain9/1 -> Mux1/2
  Fin/1 -> Demux/1
  Demux/4 -> Gain13/1
  Gain13/1 -> Mux1/4
  Mux1/1 -> Gain14/1
  Gain12/1 -> Mux1/3

== system vehicle_motion_model_final_temp/Two-Axle Vehicle/Wheels and Tires/Wheels and Tires/Tire2Veh/Subsystem2 ==
  Fin : Inport
  Demux : Demux
  Gain12 : Gain  Gain=VEH.NumberOfWheelsPerRearAxle
  Gain13 : Gain  Gain=VEH.NumberOfWheelsPerRearAxle
  Gain14 : Gain  Gain=1/2
  Gain8 : Gain  Gain=VEH.NumberOfWheelsPerFrontAxle
  Gain9 : Gain  Gain=VEH.NumberOfWheelsPerFrontAxle
  Mux1 : Mux
  Reshape : Reshape  OutputDimensionality=Column vector (2-D)
  Fout : Outport
  wires:
  Mux1/1 -> Gain14/1
  Gain13/1 -> Mux1/4
  Demux/4 -> Gain13/1
  Fin/1 -> Demux/1
  Gain9/1 -> Mux1/2
  Gain8/1 -> Mux1/1
  Gain12/1 -> Mux1/3
  Demux/2 -> Gain9/1
  Demux/1 -> Gain8/1
  Demux/3 -> Gain12/1
  Gain14/1 -> Reshape/1
  Reshape/1 -> Fout/1

== system vehicle_motion_model_final_temp/Two-Axle Vehicle/Wheels and Tires/Wheels and Tires/Tire2Veh/Subsystem3 ==
  Fin : Inport
  Demux : Demux
  Gain12 : Gain  Gain=VEH.NumberOfWheelsPerRearAxle
  Gain13 : Gain  Gain=VEH.NumberOfWheelsPerRearAxle
  Gain14 : Gain  Gain=1/2
  Gain8 : Gain  Gain=VEH.NumberOfWheelsPerFrontAxle
  Gain9 : Gain  Gain=VEH.NumberOfWheelsPerFrontAxle
  Mux1 : Mux
  Reshape : Reshape  OutputDimensionality=Column vector (2-D)
  Fout : Outport
  wires:
  Mux1/1 -> Gain14/1
  Gain13/1 -> Mux1/4
  Fin/1 -> Demux/1
  Gain9/1 -> Mux1/2
  Gain8/1 -> Mux1/1
  Gain12/1 -> Mux1/3
  Demux/2 -> Gain9/1
  Demux/1 -> Gain8/1
  Gain14/1 -> Reshape/1
  Reshape/1 -> Fout/1
  Demux/3 -> Gain12/1
  Demux/4 -> Gain13/1

== system vehicle_motion_model_final_temp/Two-Axle Vehicle/Wheels and Tires/Wheels and Tires/Tire2Veh/Wheel Angles ==
  Front : Inport
  Camber : Inport  Port=2
  Add1 : Sum
  Add2 : Sum
  Constant1 : Constant  Value=pi
  Constant2 : Constant  Value=[pi;0;pi;0].*0+[0;pi;0;pi].*.0
  Constant3 : Constant  Value=ones(1,4).*0
  Reshape : Reshape  OutputDimensionality=Row vector (2-D)
  Reshape1 : Reshape  OutputDimensionality=Row vector (2-D)
  Reshape2 : Reshape  OutputDimensionality=Row vector (2-D)
  Vector Concatenate3 : Concatenate  NumInputs=3  Mode=Multidimensional array
  Vehicle : Outport  VectorParamsAs1DForOutWhenUnconnected=off
  wires:
  Reshape/1 -> Vector Concatenate3/3
  Reshape2/1 -> Vector Concatenate3/2
  Vector Concatenate3/1 -> Vehicle/1
  Constant2/1 -> Add1/2
  Front/1 -> Add1/1
  Reshape1/1 -> Vector Concatenate3/1
  Constant3/1 -> Reshape2/1
  Add1/1 -> Reshape/1
  Camber/1 -> Add2/1
  Add2/1 -> Reshape1/1
  Constant1/1 -> Add2/2

== system vehicle_motion_model_final_temp/Two-Axle Vehicle/Wheels and Tires/Wheels and Tires/Tire2Veh/Wheel to Body Transform ==
  Forces : Inport  PortDimensions=[3,1]  Partition=on  PartitionDimension=2  PartitionWidth=1  PartitionOffset=0
  WheelAngles : Inport  Port=2  PortDimensions=[3,1]  Partition=on  PartitionDimension=2  PartitionWidth=1  PartitionOffset=0
  Demux1 : Demux  Outputs=3
  Divide1 : Product  Inputs=**  Multiplication=Matrix(*)
  For Each : ForEach  DisableCoverage=on
  Rotation Angles to Direction Cosine Matrix : sharedtransform/Rotation Angles to Direction Cosine Matrix  rotationOrder=ZYX  aMode=2
      settings: SourceProductBaseCode=AE,PW,DR,MT,UV,VE
  Selector : Selector  InputPortWidth=3  IndexOptions=Index vector (dialog)  Indices=[3 2 1]  OutputSizes=1
  Fx : Outport  ConcatenationDimension=1  VectorParamsAs1DForOutWhenUnconnected=off
  Fy : Outport  Port=2  ConcatenationDimension=1  VectorParamsAs1DForOutWhenUnconnected=off
  Fz : Outport  Port=3  ConcatenationDimension=1  VectorParamsAs1DForOutWhenUnconnected=off
  wires:
  Divide1/1 -> Demux1/1
  Demux1/1 -> Fx/1
  Demux1/2 -> Fy/1
  Demux1/3 -> Fz/1
  Rotation Angles to Direction Cosine Matrix/1 -> Divide1/1
  Forces/1 -> Divide1/2
  WheelAngles/1 -> Selector/1
  Selector/1 -> Rotation Angles to Direction Cosine Matrix/1
